simulink model "TST_Rail_PreCtlMeUn"  (R2016b)
settings: Solver=FixedStepDiscrete  StartTime=0.0  StopTime=simTime  FixedStep=sampleTime  RelTol=1e-3
values from neighbouring files (symbols this model uses):
  testCase = 1    [initTST_Rail_PreCtlMeUn_001.m]
libraries: simulink x7, UnitTest_Lib x5
settings Model: Creator=zhengjinyan  LastModifiedBy=zhengjinyan
settings DebuggingCC: SignalRangeChecking=error

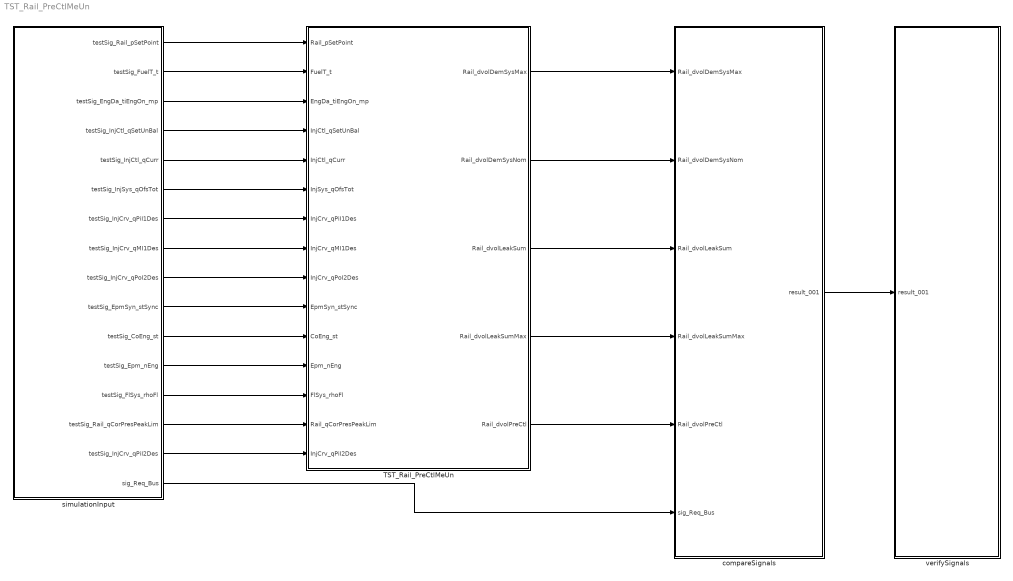
== system TST_Rail_PreCtlMeUn ==
  TST_Rail_PreCtlMeUn : Subsystem
  compareSignals : Subsystem
  simulationInput : Subsystem
  verifySignals : Subsystem
  wires:
  simulationInput/1(testSig_Rail_pSetPoint) -> TST_Rail_PreCtlMeUn/1(Rail_pSetPoint)
  simulationInput/2(testSig_FuelT_t) -> TST_Rail_PreCtlMeUn/2(FuelT_t)
  simulationInput/3(testSig_EngDa_tiEngOn_mp) -> TST_Rail_PreCtlMeUn/3(EngDa_tiEngOn_mp)
  simulationInput/4(testSig_InjCtl_qSetUnBal) -> TST_Rail_PreCtlMeUn/4(InjCtl_qSetUnBal)
  simulationInput/5(testSig_InjCtl_qCurr) -> TST_Rail_PreCtlMeUn/5(InjCtl_qCurr)
  simulationInput/6(testSig_InjSys_qOfsTot) -> TST_Rail_PreCtlMeUn/6(InjSys_qOfsTot)
  simulationInput/7(testSig_InjCrv_qPiI1Des) -> TST_Rail_PreCtlMeUn/7(InjCrv_qPiI1Des)
  simulationInput/8(testSig_InjCrv_qMI1Des) -> TST_Rail_PreCtlMeUn/8(InjCrv_qMI1Des)
  simulationInput/9(testSig_InjCrv_qPoI2Des) -> TST_Rail_PreCtlMeUn/9(InjCrv_qPoI2Des)
  simulationInput/10(testSig_EpmSyn_stSync) -> TST_Rail_PreCtlMeUn/10(EpmSyn_stSync)
  simulationInput/11(testSig_CoEng_st) -> TST_Rail_PreCtlMeUn/11(CoEng_st)
  simulationInput/12(testSig_Epm_nEng) -> TST_Rail_PreCtlMeUn/12(Epm_nEng)
  simulationInput/13(testSig_FlSys_rhoFl) -> TST_Rail_PreCtlMeUn/13(FlSys_rhoFl)
  simulationInput/14(testSig_Rail_qCorPresPeakLim) -> TST_Rail_PreCtlMeUn/14(Rail_qCorPresPeakLim)
  simulationInput/15(testSig_InjCrv_qPiI2Des) -> TST_Rail_PreCtlMeUn/15(InjCrv_qPiI2Des)
  TST_Rail_PreCtlMeUn/1(Rail_dvolDemSysMax) -> compareSignals/1(Rail_dvolDemSysMax)
  TST_Rail_PreCtlMeUn/2(Rail_dvolDemSysNom) -> compareSignals/2(Rail_dvolDemSysNom)
  TST_Rail_PreCtlMeUn/3(Rail_dvolLeakSum) -> compareSignals/3(Rail_dvolLeakSum)
  TST_Rail_PreCtlMeUn/4(Rail_dvolLeakSumMax) -> compareSignals/4(Rail_dvolLeakSumMax)
  TST_Rail_PreCtlMeUn/5(Rail_dvolPreCtl) -> compareSignals/5(Rail_dvolPreCtl)
  simulationInput/16(sig_Req_Bus) -> compareSignals/6(sig_Req_Bus)
  compareSignals/1(result_001) -> verifySignals/1(result_001)

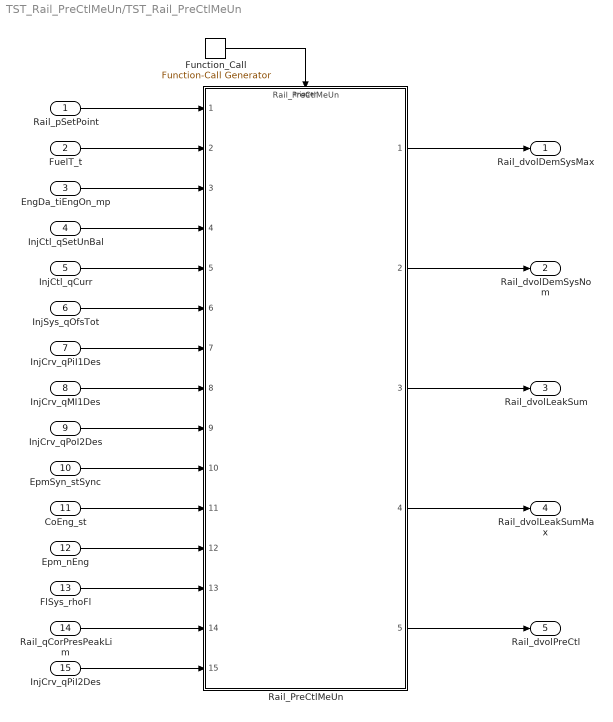
== system TST_Rail_PreCtlMeUn/TST_Rail_PreCtlMeUn ==
  Rail_pSetPoint : Inport
  FuelT_t : Inport  Port=2
  EngDa_tiEngOn_mp : Inport  Port=3
  InjCtl_qSetUnBal : Inport  Port=4
  InjCtl_qCurr : Inport  Port=5
  InjSys_qOfsTot : Inport  Port=6
  InjCrv_qPiI1Des : Inport  Port=7
  InjCrv_qMI1Des : Inport  Port=8
  InjCrv_qPoI2Des : Inport  Port=9
  EpmSyn_stSync : Inport  Port=10
  CoEng_st : Inport  Port=11
  Epm_nEng : Inport  Port=12
  FlSys_rhoFl : Inport  Port=13
  Rail_qCorPresPeakLim : Inport  Port=14
  InjCrv_qPiI2Des : Inport  Port=15
  Function_Call : simulink/Ports & Subsystems/Function-Call Generator  sample_time=sampleTime  numberOfIterations=1
  Rail_PreCtlMeUn : ModelReference  ModelNameDialog=Rail_PreCtlMeUn  SimulationMode=Normal  ModelReferenceVersion=1.60  TriggerPortName=function  TriggerPortTriggerType=function-call  TriggerPortStatesWhenEnabling=held
  Rail_dvolDemSysMax : Outport
  Rail_dvolDemSysNom : Outport  Port=2
  Rail_dvolLeakSum : Outport  Port=3
  Rail_dvolLeakSumMax : Outport  Port=4
  Rail_dvolPreCtl : Outport  Port=5
  wires:
  Function_Call/1 -> Rail_PreCtlMeUn/Trigger
  Rail_pSetPoint/1 -> Rail_PreCtlMeUn/1
  FuelT_t/1 -> Rail_PreCtlMeUn/2
  EngDa_tiEngOn_mp/1 -> Rail_PreCtlMeUn/3
  InjCtl_qSetUnBal/1 -> Rail_PreCtlMeUn/4
  InjCtl_qCurr/1 -> Rail_PreCtlMeUn/5
  InjSys_qOfsTot/1 -> Rail_PreCtlMeUn/6
  InjCrv_qPiI1Des/1 -> Rail_PreCtlMeUn/7
  InjCrv_qMI1Des/1 -> Rail_PreCtlMeUn/8
  InjCrv_qPoI2Des/1 -> Rail_PreCtlMeUn/9
  EpmSyn_stSync/1 -> Rail_PreCtlMeUn/10
  CoEng_st/1 -> Rail_PreCtlMeUn/11
  Epm_nEng/1 -> Rail_PreCtlMeUn/12
  FlSys_rhoFl/1 -> Rail_PreCtlMeUn/13
  Rail_qCorPresPeakLim/1 -> Rail_PreCtlMeUn/14
  InjCrv_qPiI2Des/1 -> Rail_PreCtlMeUn/15
  Rail_PreCtlMeUn/1 -> Rail_dvolDemSysMax/1
  Rail_PreCtlMeUn/2 -> Rail_dvolDemSysNom/1
  Rail_PreCtlMeUn/3 -> Rail_dvolLeakSum/1
  Rail_PreCtlMeUn/4 -> Rail_dvolLeakSumMax/1
  Rail_PreCtlMeUn/5 -> Rail_dvolPreCtl/1

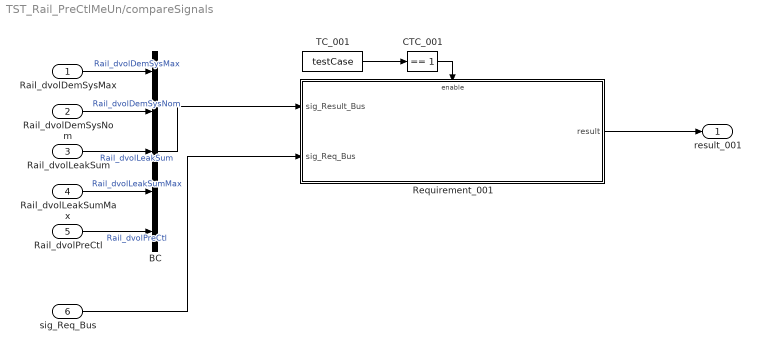
== system TST_Rail_PreCtlMeUn/compareSignals ==
  Rail_dvolDemSysMax : Inport
  Rail_dvolDemSysNom : Inport  Port=2
  Rail_dvolLeakSum : Inport  Port=3
  Rail_dvolLeakSumMax : Inport  Port=4
  Rail_dvolPreCtl : Inport  Port=5
  sig_Req_Bus : Inport  Port=6
  BC : BusCreator  Inputs=5
  CTC_001 : simulink/Logic and Bit Operations/Compare To Constant  relop===  const=1  OutDataTypeStr=boolean
  Requirement_001 : Subsystem
  TC_001 : Constant  Value=testCase
  result_001 : Outport
  wires:
  Rail_dvolDemSysMax/1 -> BC/1  "Rail_dvolDemSysMax"
  Rail_dvolDemSysNom/1 -> BC/2  "Rail_dvolDemSysNom"
  Rail_dvolLeakSum/1 -> BC/3  "Rail_dvolLeakSum"
  Rail_dvolLeakSumMax/1 -> BC/4  "Rail_dvolLeakSumMax"
  Rail_dvolPreCtl/1 -> BC/5  "Rail_dvolPreCtl"
  TC_001/1 -> CTC_001/1
  CTC_001/1 -> Requirement_001/Enable
  sig_Req_Bus/1 -> Requirement_001/2(sig_Req_Bus)
  BC/1 -> Requirement_001/1(sig_Result_Bus)
  Requirement_001/1(result) -> result_001/1

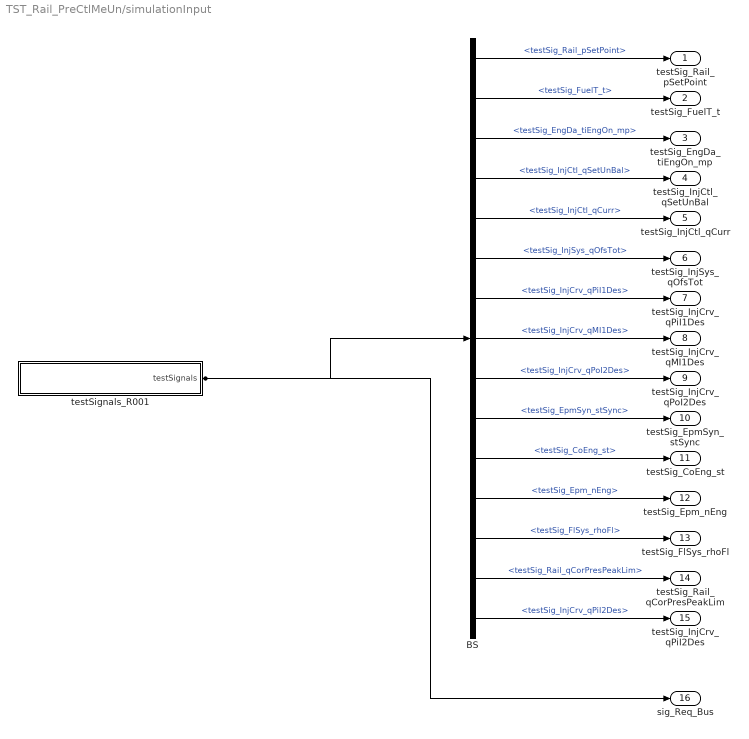
== system TST_Rail_PreCtlMeUn/simulationInput ==
  BS : BusSelector  OutputSignals=testSig_Rail_pSetPoint,testSig_FuelT_t,testSig_EngDa_tiEngOn_mp,testSig_InjCtl_qSetUnBal,testSig_InjCtl_qCurr,testSig_InjSys_qOfsTot,testSig_InjCrv_qPiI1Des,testSig_InjCrv_qMI1Des,testSig_InjCrv_qPoI2Des,testSig_EpmSyn_stSync,testSig_CoEng_st,testSig_Epm_nEng,testSig_FlSys_rhoFl,testSig_Rail_qCorPresPeakLim,testSig_InjCrv_qPiI2Des
  testSignals_R001 : Subsystem
  testSig_Rail_pSetPoint : Outport
  testSig_FuelT_t : Outport  Port=2
  testSig_EngDa_tiEngOn_mp : Outport  Port=3
  testSig_InjCtl_qSetUnBal : Outport  Port=4
  testSig_InjCtl_qCurr : Outport  Port=5
  testSig_InjSys_qOfsTot : Outport  Port=6
  testSig_InjCrv_qPiI1Des : Outport  Port=7
  testSig_InjCrv_qMI1Des : Outport  Port=8
  testSig_InjCrv_qPoI2Des : Outport  Port=9
  testSig_EpmSyn_stSync : Outport  Port=10
  testSig_CoEng_st : Outport  Port=11
  testSig_Epm_nEng : Outport  Port=12
  testSig_FlSys_rhoFl : Outport  Port=13
  testSig_Rail_qCorPresPeakLim : Outport  Port=14
  testSig_InjCrv_qPiI2Des : Outport  Port=15
  sig_Req_Bus : Outport  Port=16
  wires:
  BS/1 -> testSig_Rail_pSetPoint/1  "<testSig_Rail_pSetPoint>"
  BS/2 -> testSig_FuelT_t/1  "<testSig_FuelT_t>"
  BS/3 -> testSig_EngDa_tiEngOn_mp/1  "<testSig_EngDa_tiEngOn_mp>"
  BS/4 -> testSig_InjCtl_qSetUnBal/1  "<testSig_InjCtl_qSetUnBal>"
  BS/5 -> testSig_InjCtl_qCurr/1  "<testSig_InjCtl_qCurr>"
  BS/6 -> testSig_InjSys_qOfsTot/1  "<testSig_InjSys_qOfsTot>"
  BS/7 -> testSig_InjCrv_qPiI1Des/1  "<testSig_InjCrv_qPiI1Des>"
  BS/8 -> testSig_InjCrv_qMI1Des/1  "<testSig_InjCrv_qMI1Des>"
  BS/9 -> testSig_InjCrv_qPoI2Des/1  "<testSig_InjCrv_qPoI2Des>"
  BS/10 -> testSig_EpmSyn_stSync/1  "<testSig_EpmSyn_stSync>"
  BS/11 -> testSig_CoEng_st/1  "<testSig_CoEng_st>"
  BS/12 -> testSig_Epm_nEng/1  "<testSig_Epm_nEng>"
  BS/13 -> testSig_FlSys_rhoFl/1  "<testSig_FlSys_rhoFl>"
  BS/14 -> testSig_Rail_qCorPresPeakLim/1  "<testSig_Rail_qCorPresPeakLim>"
  BS/15 -> testSig_InjCrv_qPiI2Des/1  "<testSig_InjCrv_qPiI2Des>"
  testSignals_R001/1(testSignals) -> BS/1, sig_Req_Bus/1

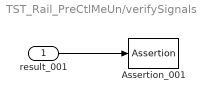
== system TST_Rail_PreCtlMeUn/verifySignals ==
  result_001 : Inport
  Assertion_001 : Assertion  Enabled=off
  wires:
  result_001/1 -> Assertion_001/1

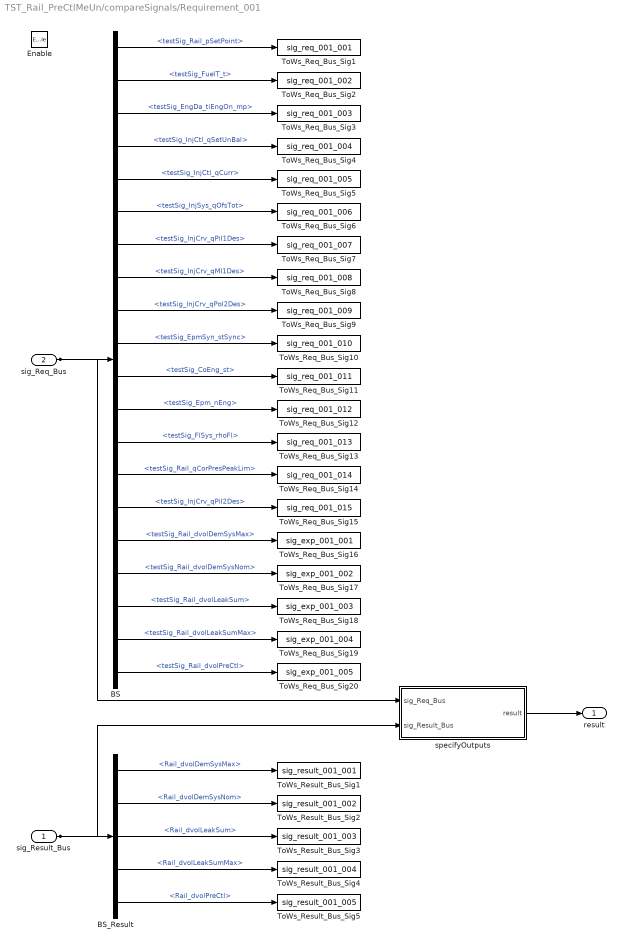
== system TST_Rail_PreCtlMeUn/compareSignals/Requirement_001 ==
  sig_Result_Bus : Inport
  sig_Req_Bus : Inport  Port=2
  Enable : EnablePort
  BS : BusSelector  OutputSignals=testSig_Rail_pSetPoint,testSig_FuelT_t,testSig_EngDa_tiEngOn_mp,testSig_InjCtl_qSetUnBal,testSig_InjCtl_qCurr,testSig_InjSys_qOfsTot,testSig_InjCrv_qPiI1Des,testSig_InjCrv_qMI1Des,testSig_InjCrv_qPoI2Des,testSig_EpmSyn_stSync,testSig_CoEng_st,testSig_Epm_nEng,testSig_FlSys_rhoFl,testSig_Rail_qCorPresPeakLim,testSig_InjCrv_qPiI2Des,testSig_Rail_dvolDemSysMax,testSig_Rail_dvolDemSysNom,testSig_Rail_dvolLeakSum,testSig_Rail_dvolLeakSumMax,testSig_Rail_dvolPreCtl
  BS_Result : BusSelector  OutputSignals=Rail_dvolDemSysMax,Rail_dvolDemSysNom,Rail_dvolLeakSum,Rail_dvolLeakSumMax,Rail_dvolPreCtl
  ToWs_Req_Bus_Sig1 : ToWorkspace  VariableName=sig_req_001_001  SaveFormat=Structure With Time
  ToWs_Req_Bus_Sig10 : ToWorkspace  VariableName=sig_req_001_010  SaveFormat=Structure With Time
  ToWs_Req_Bus_Sig11 : ToWorkspace  VariableName=sig_req_001_011  SaveFormat=Structure With Time
  ToWs_Req_Bus_Sig12 : ToWorkspace  VariableName=sig_req_001_012  SaveFormat=Structure With Time
  ToWs_Req_Bus_Sig13 : ToWorkspace  VariableName=sig_req_001_013  SaveFormat=Structure With Time
  ToWs_Req_Bus_Sig14 : ToWorkspace  VariableName=sig_req_001_014  SaveFormat=Structure With Time
  ToWs_Req_Bus_Sig15 : ToWorkspace  VariableName=sig_req_001_015  SaveFormat=Structure With Time
  ToWs_Req_Bus_Sig16 : ToWorkspace  VariableName=sig_exp_001_001  SaveFormat=Structure With Time
  ToWs_Req_Bus_Sig17 : ToWorkspace  VariableName=sig_exp_001_002  SaveFormat=Structure With Time
  ToWs_Req_Bus_Sig18 : ToWorkspace  VariableName=sig_exp_001_003  SaveFormat=Structure With Time
  ToWs_Req_Bus_Sig19 : ToWorkspace  VariableName=sig_exp_001_004  SaveFormat=Structure With Time
  ToWs_Req_Bus_Sig2 : ToWorkspace  VariableName=sig_req_001_002  SaveFormat=Structure With Time
  ToWs_Req_Bus_Sig20 : ToWorkspace  VariableName=sig_exp_001_005  SaveFormat=Structure With Time
  ToWs_Req_Bus_Sig3 : ToWorkspace  VariableName=sig_req_001_003  SaveFormat=Structure With Time
  ToWs_Req_Bus_Sig4 : ToWorkspace  VariableName=sig_req_001_004  SaveFormat=Structure With Time
  ToWs_Req_Bus_Sig5 : ToWorkspace  VariableName=sig_req_001_005  SaveFormat=Structure With Time
  ToWs_Req_Bus_Sig6 : ToWorkspace  VariableName=sig_req_001_006  SaveFormat=Structure With Time
  ToWs_Req_Bus_Sig7 : ToWorkspace  VariableName=sig_req_001_007  SaveFormat=Structure With Time
  ToWs_Req_Bus_Sig8 : ToWorkspace  VariableName=sig_req_001_008  SaveFormat=Structure With Time
  ToWs_Req_Bus_Sig9 : ToWorkspace  VariableName=sig_req_001_009  SaveFormat=Structure With Time
  ToWs_Result_Bus_Sig1 : ToWorkspace  VariableName=sig_result_001_001  SaveFormat=Structure With Time
  ToWs_Result_Bus_Sig2 : ToWorkspace  VariableName=sig_result_001_002  SaveFormat=Structure With Time
  ToWs_Result_Bus_Sig3 : ToWorkspace  VariableName=sig_result_001_003  SaveFormat=Structure With Time
  ToWs_Result_Bus_Sig4 : ToWorkspace  VariableName=sig_result_001_004  SaveFormat=Structure With Time
  ToWs_Result_Bus_Sig5 : ToWorkspace  VariableName=sig_result_001_005  SaveFormat=Structure With Time
  specifyOutputs : Subsystem
  result : Outport
  wires:
  sig_Req_Bus/1 -> BS/1, specifyOutputs/1(sig_Req_Bus)
  BS/1 -> ToWs_Req_Bus_Sig1/1  "<testSig_Rail_pSetPoint>"
  BS/2 -> ToWs_Req_Bus_Sig2/1  "<testSig_FuelT_t>"
  BS/3 -> ToWs_Req_Bus_Sig3/1  "<testSig_EngDa_tiEngOn_mp>"
  BS/4 -> ToWs_Req_Bus_Sig4/1  "<testSig_InjCtl_qSetUnBal>"
  BS/5 -> ToWs_Req_Bus_Sig5/1  "<testSig_InjCtl_qCurr>"
  BS/6 -> ToWs_Req_Bus_Sig6/1  "<testSig_InjSys_qOfsTot>"
  BS/7 -> ToWs_Req_Bus_Sig7/1  "<testSig_InjCrv_qPiI1Des>"
  BS/8 -> ToWs_Req_Bus_Sig8/1  "<testSig_InjCrv_qMI1Des>"
  BS/9 -> ToWs_Req_Bus_Sig9/1  "<testSig_InjCrv_qPoI2Des>"
  BS/10 -> ToWs_Req_Bus_Sig10/1  "<testSig_EpmSyn_stSync>"
  BS/11 -> ToWs_Req_Bus_Sig11/1  "<testSig_CoEng_st>"
  BS/12 -> ToWs_Req_Bus_Sig12/1  "<testSig_Epm_nEng>"
  BS/13 -> ToWs_Req_Bus_Sig13/1  "<testSig_FlSys_rhoFl>"
  BS/14 -> ToWs_Req_Bus_Sig14/1  "<testSig_Rail_qCorPresPeakLim>"
  BS/15 -> ToWs_Req_Bus_Sig15/1  "<testSig_InjCrv_qPiI2Des>"
  BS/16 -> ToWs_Req_Bus_Sig16/1  "<testSig_Rail_dvolDemSysMax>"
  BS/17 -> ToWs_Req_Bus_Sig17/1  "<testSig_Rail_dvolDemSysNom>"
  BS/18 -> ToWs_Req_Bus_Sig18/1  "<testSig_Rail_dvolLeakSum>"
  BS/19 -> ToWs_Req_Bus_Sig19/1  "<testSig_Rail_dvolLeakSumMax>"
  BS/20 -> ToWs_Req_Bus_Sig20/1  "<testSig_Rail_dvolPreCtl>"
  sig_Result_Bus/1 -> BS_Result/1, specifyOutputs/2(sig_Result_Bus)
  BS_Result/1 -> ToWs_Result_Bus_Sig1/1  "<Rail_dvolDemSysMax>"
  BS_Result/2 -> ToWs_Result_Bus_Sig2/1  "<Rail_dvolDemSysNom>"
  BS_Result/3 -> ToWs_Result_Bus_Sig3/1  "<Rail_dvolLeakSum>"
  BS_Result/4 -> ToWs_Result_Bus_Sig4/1  "<Rail_dvolLeakSumMax>"
  BS_Result/5 -> ToWs_Result_Bus_Sig5/1  "<Rail_dvolPreCtl>"
  specifyOutputs/1(result) -> result/1

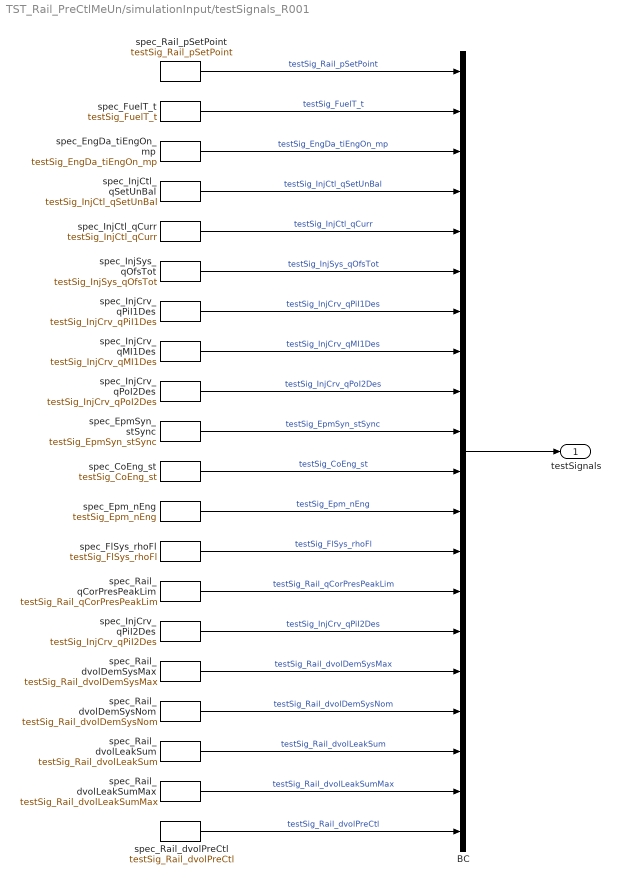
== system TST_Rail_PreCtlMeUn/simulationInput/testSignals_R001 ==
  BC : BusCreator  Inputs=20
  spec_CoEng_st : FromWorkspace  VariableName=testSig_CoEng_st  Interpolate=off  OutputAfterFinalValue=Holding final value
  spec_EngDa_tiEngOn_mp : FromWorkspace  VariableName=testSig_EngDa_tiEngOn_mp  Interpolate=off  OutputAfterFinalValue=Holding final value
  spec_EpmSyn_stSync : FromWorkspace  VariableName=testSig_EpmSyn_stSync  Interpolate=off  OutputAfterFinalValue=Holding final value
  spec_Epm_nEng : FromWorkspace  VariableName=testSig_Epm_nEng  Interpolate=off  OutputAfterFinalValue=Holding final value
  spec_FlSys_rhoFl : FromWorkspace  VariableName=testSig_FlSys_rhoFl  Interpolate=off  OutputAfterFinalValue=Holding final value
  spec_FuelT_t : FromWorkspace  VariableName=testSig_FuelT_t  Interpolate=off  OutputAfterFinalValue=Holding final value
  spec_InjCrv_qMI1Des : FromWorkspace  VariableName=testSig_InjCrv_qMI1Des  Interpolate=off  OutputAfterFinalValue=Holding final value
  spec_InjCrv_qPiI1Des : FromWorkspace  VariableName=testSig_InjCrv_qPiI1Des  Interpolate=off  OutputAfterFinalValue=Holding final value
  spec_InjCrv_qPiI2Des : FromWorkspace  VariableName=testSig_InjCrv_qPiI2Des  Interpolate=off  OutputAfterFinalValue=Holding final value
  spec_InjCrv_qPoI2Des : FromWorkspace  VariableName=testSig_InjCrv_qPoI2Des  Interpolate=off  OutputAfterFinalValue=Holding final value
  spec_InjCtl_qCurr : FromWorkspace  VariableName=testSig_InjCtl_qCurr  Interpolate=off  OutputAfterFinalValue=Holding final value
  spec_InjCtl_qSetUnBal : FromWorkspace  VariableName=testSig_InjCtl_qSetUnBal  Interpolate=off  OutputAfterFinalValue=Holding final value
  spec_InjSys_qOfsTot : FromWorkspace  VariableName=testSig_InjSys_qOfsTot  Interpolate=off  OutputAfterFinalValue=Holding final value
  spec_Rail_dvolDemSysMax : FromWorkspace  VariableName=testSig_Rail_dvolDemSysMax  Interpolate=off  OutputAfterFinalValue=Holding final value
  spec_Rail_dvolDemSysNom : FromWorkspace  VariableName=testSig_Rail_dvolDemSysNom  Interpolate=off  OutputAfterFinalValue=Holding final value
  spec_Rail_dvolLeakSum : FromWorkspace  VariableName=testSig_Rail_dvolLeakSum  Interpolate=off  OutputAfterFinalValue=Holding final value
  spec_Rail_dvolLeakSumMax : FromWorkspace  VariableName=testSig_Rail_dvolLeakSumMax  Interpolate=off  OutputAfterFinalValue=Holding final value
  spec_Rail_dvolPreCtl : FromWorkspace  VariableName=testSig_Rail_dvolPreCtl  Interpolate=off  OutputAfterFinalValue=Holding final value
  spec_Rail_pSetPoint : FromWorkspace  VariableName=testSig_Rail_pSetPoint  Interpolate=off  OutputAfterFinalValue=Holding final value
  spec_Rail_qCorPresPeakLim : FromWorkspace  VariableName=testSig_Rail_qCorPresPeakLim  Interpolate=off  OutputAfterFinalValue=Holding final value
  testSignals : Outport
  wires:
  BC/1 -> testSignals/1
  spec_Rail_pSetPoint/1 -> BC/1  "testSig_Rail_pSetPoint"
  spec_FuelT_t/1 -> BC/2  "testSig_FuelT_t"
  spec_EngDa_tiEngOn_mp/1 -> BC/3  "testSig_EngDa_tiEngOn_mp"
  spec_InjCtl_qSetUnBal/1 -> BC/4  "testSig_InjCtl_qSetUnBal"
  spec_InjCtl_qCurr/1 -> BC/5  "testSig_InjCtl_qCurr"
  spec_InjSys_qOfsTot/1 -> BC/6  "testSig_InjSys_qOfsTot"
  spec_InjCrv_qPiI1Des/1 -> BC/7  "testSig_InjCrv_qPiI1Des"
  spec_InjCrv_qMI1Des/1 -> BC/8  "testSig_InjCrv_qMI1Des"
  spec_InjCrv_qPoI2Des/1 -> BC/9  "testSig_InjCrv_qPoI2Des"
  spec_EpmSyn_stSync/1 -> BC/10  "testSig_EpmSyn_stSync"
  spec_CoEng_st/1 -> BC/11  "testSig_CoEng_st"
  spec_Epm_nEng/1 -> BC/12  "testSig_Epm_nEng"
  spec_FlSys_rhoFl/1 -> BC/13  "testSig_FlSys_rhoFl"
  spec_Rail_qCorPresPeakLim/1 -> BC/14  "testSig_Rail_qCorPresPeakLim"
  spec_InjCrv_qPiI2Des/1 -> BC/15  "testSig_InjCrv_qPiI2Des"
  spec_Rail_dvolDemSysMax/1 -> BC/16  "testSig_Rail_dvolDemSysMax"
  spec_Rail_dvolDemSysNom/1 -> BC/17  "testSig_Rail_dvolDemSysNom"
  spec_Rail_dvolLeakSum/1 -> BC/18  "testSig_Rail_dvolLeakSum"
  spec_Rail_dvolLeakSumMax/1 -> BC/19  "testSig_Rail_dvolLeakSumMax"
  spec_Rail_dvolPreCtl/1 -> BC/20  "testSig_Rail_dvolPreCtl"

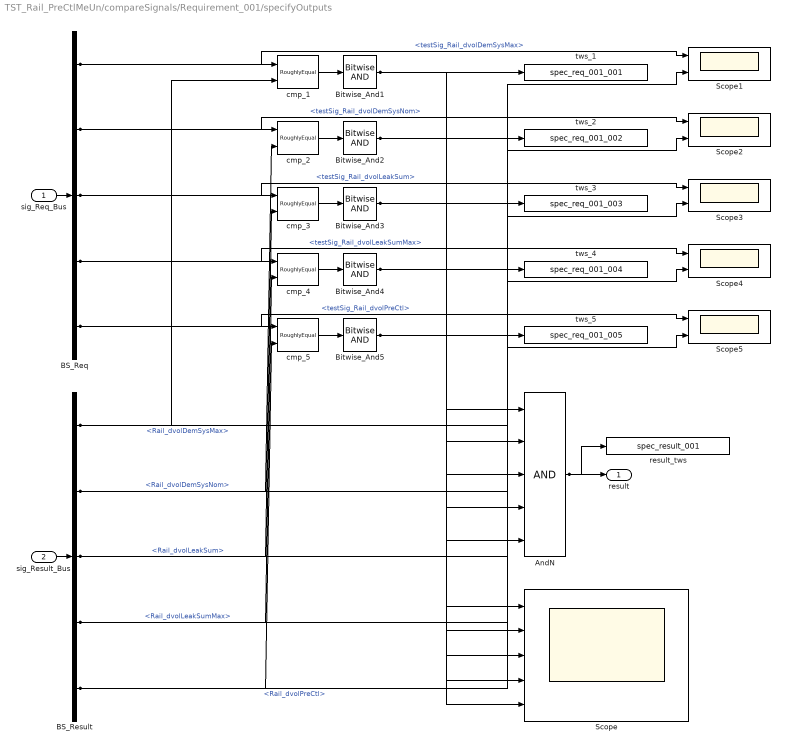
== system TST_Rail_PreCtlMeUn/compareSignals/Requirement_001/specifyOutputs ==
  sig_Req_Bus : Inport
  sig_Result_Bus : Inport  Port=2
  AndN : Logic  Inputs=5
  BS_Req : BusSelector  OutputSignals=testSig_Rail_dvolDemSysMax,testSig_Rail_dvolDemSysNom,testSig_Rail_dvolLeakSum,testSig_Rail_dvolLeakSumMax,testSig_Rail_dvolPreCtl
  BS_Result : BusSelector  OutputSignals=Rail_dvolDemSysMax,Rail_dvolDemSysNom,Rail_dvolLeakSum,Rail_dvolLeakSumMax,Rail_dvolPreCtl
  Bitwise_And{1..5} (5 alike) : simulink/Logic and Bit Operations/Bitwise Operator  logicop=AND  UseBitMask=off  BitMask=bin2dec('11011001')  BitMaskRealWorld=Stored Integer
  Scope : Scope  NumInputPorts=5
  Scope{1..5} (5 alike) : Scope  NumInputPorts=2
  cmp_{1..5} (5 alike) : UnitTest_Lib/RoughlyEqual  slope=0.1
  result_tws : ToWorkspace  VariableName=spec_result_001
  tws_1 : ToWorkspace  VariableName=spec_req_001_001
  tws_2 : ToWorkspace  VariableName=spec_req_001_002
  tws_3 : ToWorkspace  VariableName=spec_req_001_003
  tws_4 : ToWorkspace  VariableName=spec_req_001_004
  tws_5 : ToWorkspace  VariableName=spec_req_001_005
  result : Outport
  wires:
  sig_Req_Bus/1 -> BS_Req/1
  sig_Result_Bus/1 -> BS_Result/1
  AndN/1 -> result/1, result_tws/1
  BS_Req/1 -> cmp_1/1, Scope1/1  "<testSig_Rail_dvolDemSysMax>"
  BS_Result/1 -> cmp_1/2, Scope1/2  "<Rail_dvolDemSysMax>"
  cmp_1/1 -> Bitwise_And1/1
  Bitwise_And1/1 -> tws_1/1, AndN/1, Scope/1
  BS_Req/2 -> cmp_2/1, Scope2/1  "<testSig_Rail_dvolDemSysNom>"
  BS_Result/2 -> cmp_2/2, Scope2/2  "<Rail_dvolDemSysNom>"
  cmp_2/1 -> Bitwise_And2/1
  Bitwise_And2/1 -> tws_2/1, AndN/2, Scope/2
  BS_Req/3 -> cmp_3/1, Scope3/1  "<testSig_Rail_dvolLeakSum>"
  BS_Result/3 -> cmp_3/2, Scope3/2  "<Rail_dvolLeakSum>"
  cmp_3/1 -> Bitwise_And3/1
  Bitwise_And3/1 -> tws_3/1, AndN/3, Scope/3
  BS_Req/4 -> cmp_4/1, Scope4/1  "<testSig_Rail_dvolLeakSumMax>"
  BS_Result/4 -> cmp_4/2, Scope4/2  "<Rail_dvolLeakSumMax>"
  cmp_4/1 -> Bitwise_And4/1
  Bitwise_And4/1 -> tws_4/1, AndN/4, Scope/4
  BS_Req/5 -> cmp_5/1, Scope5/1  "<testSig_Rail_dvolPreCtl>"
  BS_Result/5 -> cmp_5/2, Scope5/2  "<Rail_dvolPreCtl>"
  cmp_5/1 -> Bitwise_And5/1
  Bitwise_And5/1 -> tws_5/1, AndN/5, Scope/5
